simulink model "EV_dcm_sol"  (Simulink 7.1)
settings: Solver=ode4  StartTime=SIM.t_min  StopTime=SIM.t_simul  FixedStep=1e-3  RelTol=1e-3
undefined symbols (not defined in the file): BATp, CHAi, CHAp, CHp, EMi, EMp, MTp, RDp
libraries: simulink x1
settings Model: Creator=Tony  LastModifiedBy=Alain  ExtModeTrigMode=oneshot  ExtModeArmWhenConnect=off
settings DataIOCC: LimitDataPoints=off  SignalLoggingName=sigsOut
settings OptimizationCC: BooleanDataType=off  InitFltsAndDblsToZero=off
settings DebuggingCC: SaveWithParameterizedLinksMsg=none  SignalResolutionControl=TryResolveAllWithWarning  SolverPrmCheckMsg=none  MultiTaskDSMMsg=warning  MultiTaskCondExecSysMsg=none  StrictBusMsg=None
settings HardwareCC: TargetUnknown=on
settings RTWCC: IncludeERTFirstTime=on

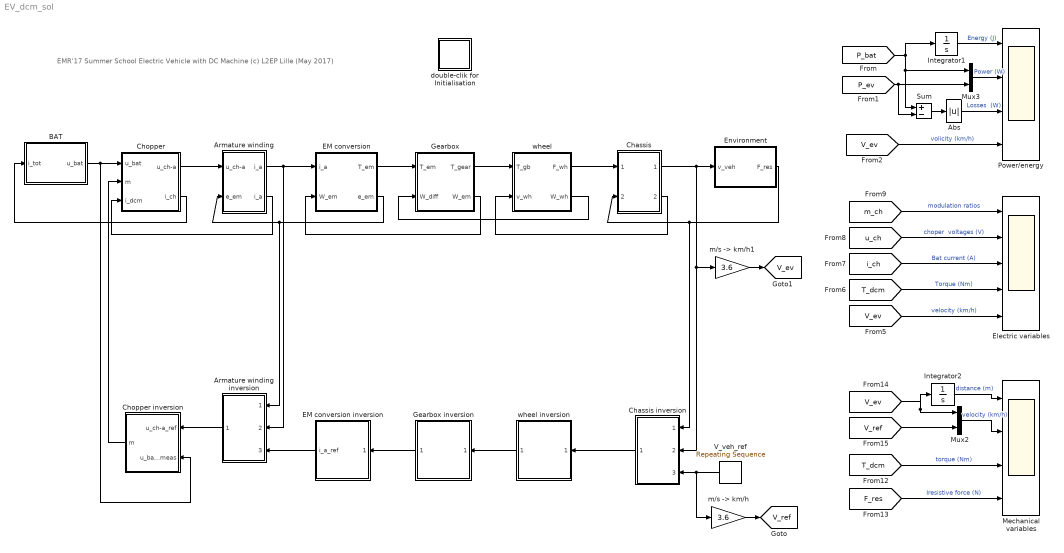
== system EV_dcm_sol ==
  note: EMR'17 Summer School
      | Electric Vehicle with DC Machine
      | (c) L2EP Lille (May 2017)
  Abs : Abs  OutDataType=sfix(16)  OutScaling=2^0
  Armature winding : Subsystem  AncestorBlock=simulink/REM/EA
      mask Type: CM
      mask Display: plot(0,0,100,100,[10,10,90,90,10],[90,10,10,90,90], [10,90],[10,90])
  Armature winding inversion : Subsystem  Orientation=left  AncestorBlock=simulink/SMC/Asservissement Correcteur IP
      mask Display: plot(0,0,100,100, [10,30,90,70,10,90],[90,10,10,90,90,10])
  BAT : Subsystem  AncestorBlock=simulink/REM/SE
      mask Display:
      | plot(0,0,100,100, 1.2*[50,57.68,60.77,63.08,64.97,66.58,68,69.26,70.4, 	71.42,72.36,78.28,80,78.28,72.36,71.42,70.4, 	69.26,68,66.58,64.97,63.08,60.77,57.68,50,42.32, 	39.23,36.92,35.03,33.42,32,30.74,29.6,28.58, 	27.64,21.72,20,21.72,27.64,28.58,29.6,30.74,32, 	33.42,35.03,36.92,39.23,42.32,50]-10, 1.2*[20,21,22,23,24,25,26,27,28,29,30,40,50,60,70,71,72, 	73,74,75,76,77,78,79,80,79,78,77,76,75,74,73,72, 	71,70,60,50,40,30,29,28,27,26,25,24,23,22,21,20]-10)
      | disp('BAT')
  Chassis : Subsystem  AncestorBlock=simulink/REM/EA
      mask Type: CM
      mask Display: plot(0,0,100,100,[10,10,90,90,10],[90,10,10,90,90], [10,90],[10,90])
  Chassis inversion : Subsystem  Orientation=left  AncestorBlock=simulink/SMC/Asservissement Correcteur IP
      mask Display: plot(0,0,100,100, [10,30,90,70,10,90],[90,10,10,90,90,10])
  Chopper : Subsystem  AncestorBlock=simulink/REM/EC Elec
      mask Type: Hacheur
      mask Display: plot(0,0,100,100,[10,10,90,90,10],[90,10,10,90,90])
  Chopper inversion : Subsystem  Orientation=left  AncestorBlock=simulink/SMC/Inversion EC avec mesure
      mask Display: plot(0,0,100,100,[10,30,90,70,10],[90,10,10,90,90])
  EM conversion : Subsystem  AncestorBlock=simulink/REM/EC EM
      mask Display: plot(0,0,100,100, 1.4*[50,57.68,60.77,63.08,64.97,66.58,68,69.26,70.4, 	71.42,72.36,78.28,80,78.28,72.36,71.42,70.4, 	69.26,68,66.58,64.97,63.08,60.77,57.68,50,42.32, 	39.23,36.92,35.03,33.42,32,30.74,29.6,28.58, 	27.64,21.72,20,21.72,27.64,28.58,29.6,30.74,32, 	33.42,35.03,36.92,39.23,42.32,50]-20, 1.4*[20,21,22,23,24,25,26,27,28,29,30,40,50,60,70,71,72, 	73,74,75,76,77,78,79,80,79,78,77,76,75,74,73,72, 	71,70,60,50,40,30,29,28,27,26,25,24,23,22,21,20]-20)
  EM conversion inversion : Subsystem  Orientation=left  AncestorBlock=simulink/SMC/Inversion EC avec mesure
      mask Display: plot(0,0,100,100,[10,30,90,70,10],[90,10,10,90,90])
  Electric variables : Scope  NumInputPorts=5
      settings: TimeRange=200  YMin=-0.5~-100~-20~-100~0  YMax=1~400~60~150~60  SaveName=ScopeData3  Decimation=10
  Environment : Subsystem  AncestorBlock=simulink/REM/SE
      mask Display:
      | plot(0,0,100,100, 1.2*[50,57.68,60.77,63.08,64.97,66.58,68,69.26,70.4, 	71.42,72.36,78.28,80,78.28,72.36,71.42,70.4, 	69.26,68,66.58,64.97,63.08,60.77,57.68,50,42.32, 	39.23,36.92,35.03,33.42,32,30.74,29.6,28.58, 	27.64,21.72,20,21.72,27.64,28.58,29.6,30.74,32, 	33.42,35.03,36.92,39.23,42.32,50]-10, 1.2*[20,21,22,23,24,25,26,27,28,29,30,40,50,60,70,71,72, 	73,74,75,76,77,78,79,80,79,78,77,76,75,74,73,72, 	71,70,60,50,40,30,29,28,27,26,25,24,23,22,21,20]-10)
      | disp('ROAD')
  Gearbox : Subsystem  AncestorBlock=simulink/REM/EC Elec
      mask Type: Hacheur
      mask Display: plot(0,0,100,100,[10,10,90,90,10],[90,10,10,90,90])
  Gearbox inversion : Subsystem  Orientation=left  AncestorBlock=simulink/SMC/Inversion EC avec mesure
      mask Display: plot(0,0,100,100,[10,30,90,70,10],[90,10,10,90,90])
  Integrator1 : Integrator
  Integrator2 : Integrator
  Mechanical variables : Scope  NumInputPorts=4
      settings: TimeRange=200  YMin=-1000~0~-100~0  YMax=4000~60~150~200  SaveName=ScopeData5  Decimation=10
  Mux2 : Mux  Inputs=2
  Mux3 : Mux  Inputs=2
  Power/energy : Scope  NumInputPorts=4
      settings: TimeRange=200  YMin=0~-10000~0~0  YMax=500000~20000~8000~60  Decimation=10
  Sum : Sum  Inputs=+-  OutDataType=sfix(16)  OutScaling=2^0  SaturateOnIntegerOverflow=on  InputSameDT=on  OutDataTypeStr=Inherit: Same as first input
  V_veh_ref : simulink/Sources/Repeating Sequence  Orientation=left  SystemSampleTime=-1  rep_seq_t=CYCL.time_ECE  rep_seq_y=CYCL.velocity_ECE
  double-clik for Initialisation : Subsystem
      settings: OpenFcn=init_EV_dcm_sol
      mask Type: Initialisation
      mask Display: disp('INIT')
  "m/s -> km/h" : Gain  Gain=3.6
  "m/s -> km/h1" : Gain  Gain=3.6
  wheel : Subsystem  AncestorBlock=simulink/REM/EC Elec
      mask Type: Hacheur
      mask Display: plot(0,0,100,100,[10,10,90,90,10],[90,10,10,90,90])
  wheel inversion : Subsystem  Orientation=left  AncestorBlock=simulink/SMC/Inversion EC avec mesure
      mask Display: plot(0,0,100,100,[10,30,90,70,10],[90,10,10,90,90])
  tag scope: V_ev=global, V_ref=global
  wires:
  BAT/1(u_bat) -> Chopper/1(u_bat), Chopper inversion/2(u_bat_meas)
  Chopper/2(i_ch) -> BAT/1(i_tot)
  Armature winding/2(i_a) -> Chopper/3(i_dcm)
  EM conversion/1(T_em) -> Gearbox/1(T_em)
  EM conversion/2(e_em) -> Armature winding/2(e_em), Armature winding inversion/1(e_em_meas)
  Gearbox/2(W_em) -> EM conversion/2(W_em)
  Chassis/1("v_veh ") -> Environment/1(v_veh), Chassis inversion/2(v_veh_meas), "m/s -> km/h1"/1
  V_veh_ref/1 -> Chassis inversion/3(v_veh_ref), "m/s -> km/h"/1
  Chassis inversion/1(F_veh_ref) -> wheel inversion/1(F_rwh_ref)
  wheel inversion/1(T_rdiff_ref) -> Gearbox inversion/1(T_gear_ref)
  Gearbox inversion/1(T_em_ref) -> EM conversion inversion/1(T_em_ref)
  Armature winding/1("i_a ") -> EM conversion/1(i_a), Armature winding inversion/2(i_a_meas)
  EM conversion inversion/1(i_a_ref) -> Armature winding inversion/3(i_a_ref)
  Chopper/1(u_ch-a) -> Armature winding/1(u_ch-a)
  Armature winding inversion/1(u_ch-a_ref) -> Chopper inversion/1(u_ch-a_ref)
  Chopper inversion/1(m) -> Chopper/2(m)
  [V_ev] -> Mux2/1, Integrator2/1
  [V_ref] -> Mux2/2
  Mux2/1 -> Mechanical variables/2  "velocity (km/h)"
  Integrator2/1 -> Mechanical variables/1  "distance (m)"
  [F_res] -> Mechanical variables/4  "Iresistive force (N)"
  [T_dcm] -> Mechanical variables/3  "torque (Nm)"
  "m/s -> km/h"/1 -> [V_ref]
  "m/s -> km/h1"/1 -> [V_ev]
  Sum/1 -> Abs/1
  [P_bat] -> Mux3/1, Sum/1, Integrator1/1
  [P_ev] -> Mux3/2, Sum/2
  [V_ev] -> Power/energy/4  "volicity (km/h)"
  Abs/1 -> Power/energy/3  "Losses  (W)"
  Mux3/1 -> Power/energy/2  "Power (W)"
  Integrator1/1 -> Power/energy/1  "Energy (J)"
  [V_ev] -> Electric variables/5  "velocity (km/h)"
  [T_dcm] -> Electric variables/4  "Torque (Nm)"
  [i_ch] -> Electric variables/3  "Bat current (A)"
  [u_ch] -> Electric variables/2  "choper  voltages (V)"
  [m_ch] -> Electric variables/1  "modulation ratios"
  Gearbox/1(T_gear) -> wheel/1(T_gb)
  wheel/1(F_wh) -> Chassis/1(F_wh)
  Chassis/2(v_veh) -> wheel/2(v_wh)
  wheel/2(W_wh) -> Gearbox/2(W_diff)
  Environment/1(F_res) -> Chassis/2(F_res), Chassis inversion/1(F_res_meas)

== system EV_dcm_sol/Armature winding ==
  u_ch-a : Inport
  e_em : Inport  Orientation=left  Port=2
  +/- : Sum  Inputs=+-  SaturateOnIntegerOverflow=on  InputSameDT=on  OutDataTypeStr=Inherit: Same as first input
  Transfer Fcn : TransferFcn  Numerator=[EMp.K_arm]  Denominator=[EMp.T_arm 1]
  "i_a " : Outport  InitialOutput=0
  i_a : Outport  Orientation=left  Port=2  InitialOutput=0
  wires:
  u_ch-a/1 -> +/-/1
  Transfer Fcn/1 -> i_a/1, "i_a "/1
  e_em/1 -> +/-/2
  +/-/1 -> Transfer Fcn/1

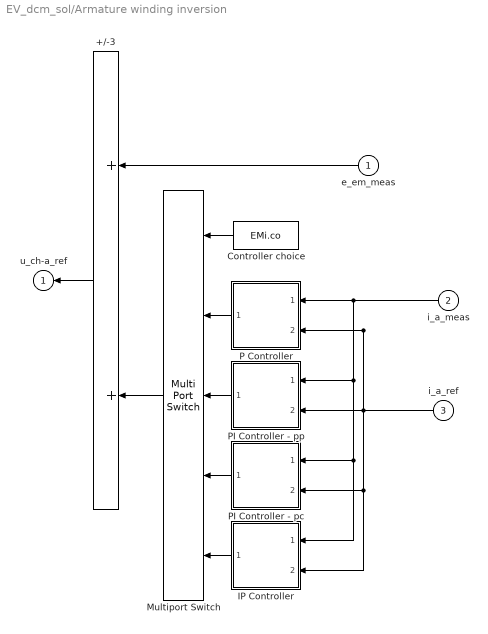
== system EV_dcm_sol/Armature winding inversion ==
  e_em_meas : Inport  Orientation=left
  i_a_meas : Inport  Orientation=left  Port=2
  i_a_ref : Inport  Orientation=left  Port=3
  +/-3 : Sum  Orientation=left  SaturateOnIntegerOverflow=on  InputSameDT=on  OutDataTypeStr=Inherit: Same as first input
  Controller choice : Constant  Orientation=left  Value=EMi.co
  IP Controller : Subsystem  Orientation=left
  Multiport Switch : MultiPortSwitch  Orientation=left  Inputs=4
  P Controller : Subsystem  Orientation=left
  PI Controller - pc : Subsystem  Orientation=left
  PI Controller - pp : Subsystem  Orientation=left
  u_ch-a_ref : Outport  Orientation=left  InitialOutput=0
  wires:
  Controller choice/1 -> Multiport Switch/1
  i_a_ref/1 -> PI Controller - pp/2(i_a_ref), PI Controller - pc/2(i_a_ref), IP Controller/2(i_a_ref), P Controller/2(i_a_ref)
  i_a_meas/1 -> PI Controller - pp/1(i_a_meas), PI Controller - pc/1(i_a_meas), IP Controller/1(i_a_meas), P Controller/1(i_a_meas)
  PI Controller - pc/1(u_ch-a_ref') -> Multiport Switch/4
  PI Controller - pp/1(u_ch-a_ref') -> Multiport Switch/3
  P Controller/1(u_ch-a_ref') -> Multiport Switch/2
  +/-3/1 -> u_ch-a_ref/1
  IP Controller/1(u_ch-a_ref') -> Multiport Switch/5
  Multiport Switch/1 -> +/-3/2
  e_em_meas/1 -> +/-3/1

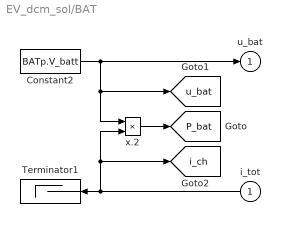
== system EV_dcm_sol/BAT ==
  i_tot : Inport  Orientation=left
  Constant2 : Constant  Value=BATp.V_batt
  Terminator1 : Terminator
  x.2 : Product  OutDataType=sfix(16)  OutScaling=2^0  SaturateOnIntegerOverflow=on  InputSameDT=on  OutDataTypeStr=Inherit: Same as first input
  u_bat : Outport  InitialOutput=0
  tag scope: P_bat=global, i_ch=global, u_bat=global
  wires:
  Constant2/1 -> u_bat/1, x.2/1, [u_bat]
  i_tot/1 -> Terminator1/1, x.2/2, [i_ch]
  x.2/1 -> [P_bat]

== system EV_dcm_sol/Chassis ==
  F_wh : Inport
  F_res : Inport  Orientation=left  Port=2
  +/- : Sum  Inputs=+-  SaturateOnIntegerOverflow=on  InputSameDT=on  OutDataTypeStr=Inherit: Same as first input
  Transfer Fcn : TransferFcn  Numerator=[CHAp.K_eq]  Denominator=[1 0]
  "v_veh " : Outport  InitialOutput=0
  v_veh : Outport  Orientation=left  Port=2  InitialOutput=0
  wires:
  +/-/1 -> Transfer Fcn/1
  F_res/1 -> +/-/2
  Transfer Fcn/1 -> "v_veh "/1, v_veh/1
  F_wh/1 -> +/-/1

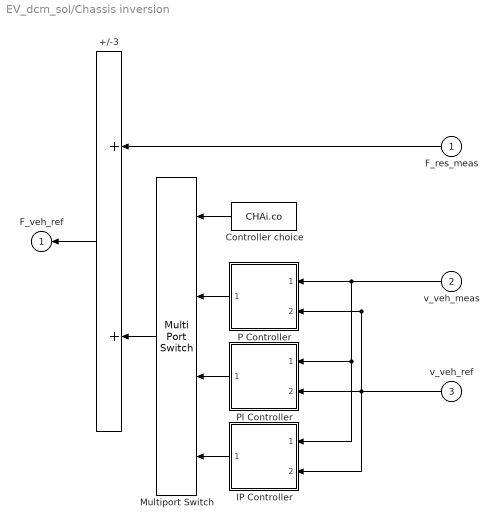
== system EV_dcm_sol/Chassis inversion ==
  F_res_meas : Inport  Orientation=left
  v_veh_meas : Inport  Orientation=left  Port=2
  v_veh_ref : Inport  Orientation=left  Port=3
  +/-3 : Sum  Orientation=left  SaturateOnIntegerOverflow=on  InputSameDT=on  OutDataTypeStr=Inherit: Same as first input
  Controller choice : Constant  Orientation=left  Value=CHAi.co
  IP Controller : Subsystem  Orientation=left
  Multiport Switch : MultiPortSwitch  Orientation=left
  P Controller : Subsystem  Orientation=left
  PI Controller : Subsystem  Orientation=left
  F_veh_ref : Outport  Orientation=left  InitialOutput=0
  wires:
  +/-3/1 -> F_veh_ref/1
  F_res_meas/1 -> +/-3/1
  Multiport Switch/1 -> +/-3/2
  P Controller/1(F_veh_ref') -> Multiport Switch/2
  PI Controller/1(F_veh_ref') -> Multiport Switch/3
  IP Controller/1(F_veh_ref') -> Multiport Switch/4
  v_veh_meas/1 -> P Controller/1(v_veh_meas), PI Controller/1(v_veh_meas), IP Controller/1(v_veh_meas)
  v_veh_ref/1 -> P Controller/2(v_veh_ref), PI Controller/2(v_veh_ref), IP Controller/2(v_veh_ref)
  Controller choice/1 -> Multiport Switch/1

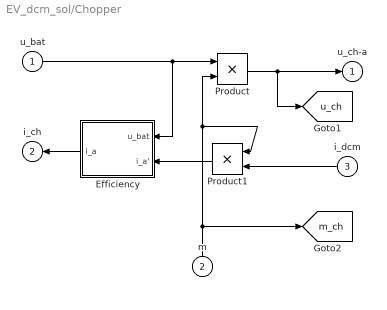
== system EV_dcm_sol/Chopper ==
  u_bat : Inport
  m : Inport  Orientation=up  Port=2
  i_dcm : Inport  Orientation=left  Port=3
  Efficiency : Subsystem  Orientation=left
  Product : Product  RndMeth=Zero
  Product1 : Product  Orientation=left  RndMeth=Zero
  u_ch-a : Outport  InitialOutput=0
  i_ch : Outport  Orientation=left  Port=2  InitialOutput=0
  tag scope: m_ch=global, u_ch=global
  wires:
  Product/1 -> u_ch-a/1, [u_ch]
  i_dcm/1 -> Product1/2
  m/1 -> Product1/1, Product/2, [m_ch]
  u_bat/1 -> Product/1, Efficiency/1(u_bat)
  Product1/1 -> Efficiency/2(i_a')
  Efficiency/1(i_a) -> i_ch/1

== system EV_dcm_sol/Chopper inversion ==
  u_ch-a_ref : Inport  Orientation=left
  u_bat_meas : Inport  Orientation=left  Port=2
  Divide : Product  Orientation=left  Inputs=*/
  Saturation : Saturate  Orientation=left  UpperLimit=1  LowerLimit=-1
  m : Outport  Orientation=left  InitialOutput=0
  wires:
  Divide/1 -> Saturation/1
  u_ch-a_ref/1 -> Divide/1
  u_bat_meas/1 -> Divide/2
  Saturation/1 -> m/1

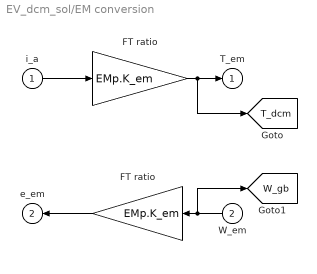
== system EV_dcm_sol/EM conversion ==
  i_a : Inport
  W_em : Inport  Orientation=left  Port=2
  FT ratio : Gain  Gain=EMp.K_em
  "FT ratio " : Gain  Orientation=left  Gain=EMp.K_em
  T_em : Outport  InitialOutput=0
  e_em : Outport  Orientation=left  Port=2  InitialOutput=0
  tag scope: T_dcm=global, W_gb=global
  wires:
  "FT ratio "/1 -> e_em/1
  i_a/1 -> FT ratio/1
  FT ratio/1 -> T_em/1, [T_dcm]
  W_em/1 -> "FT ratio "/1, [W_gb]

== system EV_dcm_sol/EM conversion inversion ==
  T_em_ref : Inport  Orientation=left
  "1/FT ratio " : Gain  Orientation=left  Gain=1/EMp.K_em
  i_a_ref : Outport  Orientation=left  InitialOutput=0
  wires:
  "1/FT ratio "/1 -> i_a_ref/1
  T_em_ref/1 -> "1/FT ratio "/1

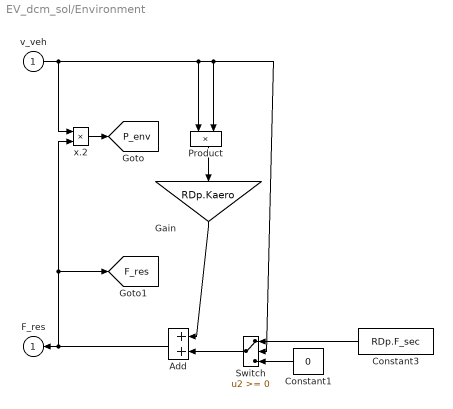
== system EV_dcm_sol/Environment ==
  v_veh : Inport
  Add : Sum  Orientation=left
  Constant1 : Constant  Orientation=left  Value=0
  Constant3 : Constant  Orientation=left  Value=RDp.F_sec
  Gain : Gain  Orientation=down  Gain=RDp.Kaero  SaturateOnIntegerOverflow=on  OutDataTypeStr=Inherit: Same as input  ParamDataTypeStr=Inherit: Same as input
  Product : Product  Orientation=down  SaturateOnIntegerOverflow=on  InputSameDT=on  OutDataTypeStr=Inherit: Same as first input
  Switch : Switch  Orientation=left
  x.2 : Product  OutDataType=sfix(16)  OutScaling=2^0  SaturateOnIntegerOverflow=on  InputSameDT=on  OutDataTypeStr=Inherit: Same as first input
  F_res : Outport  Orientation=left  InitialOutput=0
  tag scope: F_res=global, P_env=global
  wires:
  Product/1 -> Gain/1
  Gain/1 -> Add/1
  Add/1 -> F_res/1, x.2/2, [F_res]
  Constant1/1 -> Switch/3
  Constant3/1 -> Switch/1
  Switch/1 -> Add/2
  v_veh/1 -> Switch/2, Product/2, Product/1, x.2/1
  x.2/1 -> [P_env]

== system EV_dcm_sol/Gearbox ==
  T_em : Inport
  W_diff : Inport  Orientation=left  Port=2
  Efficiency : Subsystem
  FT ratio : Gain  Gain=MTp.K_gear
  "FT ratio " : Gain  Orientation=left  Gain=MTp.K_gear
  T_gear : Outport  InitialOutput=0
  W_em : Outport  Orientation=left  Port=2  InitialOutput=0
  wires:
  Efficiency/1(T_gear') -> FT ratio/1
  "FT ratio "/1 -> Efficiency/2(W_em), W_em/1
  T_em/1 -> Efficiency/1(T_em)
  FT ratio/1 -> T_gear/1
  W_diff/1 -> "FT ratio "/1

== system EV_dcm_sol/Gearbox inversion ==
  T_gear_ref : Inport  Orientation=left
  "1/FT ratio " : Gain  Orientation=left  Gain=1/MTp.K_gear
  T_em_ref : Outport  Orientation=left  InitialOutput=0
  wires:
  T_gear_ref/1 -> "1/FT ratio "/1
  "1/FT ratio "/1 -> T_em_ref/1

== system EV_dcm_sol/double-clik for Initialisation ==

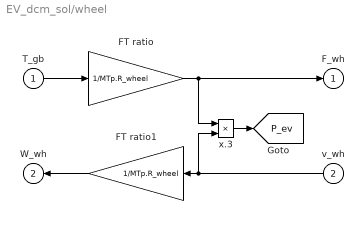
== system EV_dcm_sol/wheel ==
  T_gb : Inport
  v_wh : Inport  Orientation=left  Port=2
  FT ratio : Gain  Gain=1/MTp.R_wheel
  FT ratio1 : Gain  Orientation=left  Gain=1/MTp.R_wheel
  x.3 : Product  OutDataType=sfix(16)  OutScaling=2^0  SaturateOnIntegerOverflow=on  InputSameDT=on  OutDataTypeStr=Inherit: Same as first input
  F_wh : Outport  InitialOutput=0
  W_wh : Outport  Orientation=left  Port=2  InitialOutput=0
  tag scope: P_ev=global
  wires:
  v_wh/1 -> FT ratio1/1, x.3/2
  FT ratio/1 -> F_wh/1, x.3/1
  T_gb/1 -> FT ratio/1
  FT ratio1/1 -> W_wh/1
  x.3/1 -> [P_ev]

== system EV_dcm_sol/wheel inversion ==
  F_rwh_ref : Inport  Orientation=left
  "1/FT ratio " : Gain  Orientation=left  Gain=MTp.R_wheel
  T_rdiff_ref : Outport  Orientation=left  InitialOutput=0
  wires:
  "1/FT ratio "/1 -> T_rdiff_ref/1
  F_rwh_ref/1 -> "1/FT ratio "/1

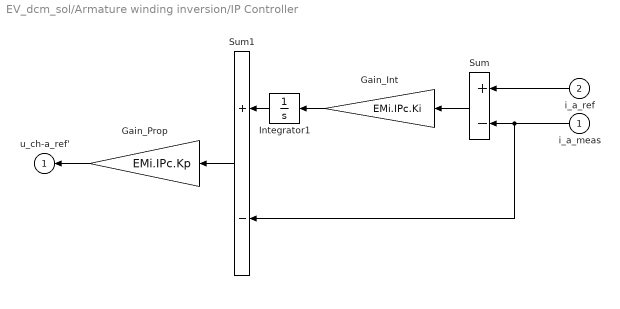
== system EV_dcm_sol/Armature winding inversion/IP Controller ==
  i_a_meas : Inport  Orientation=left
  i_a_ref : Inport  Orientation=left  Port=2
  Gain_Int : Gain  Orientation=left  Gain=EMi.IPc.Ki  SaturateOnIntegerOverflow=on  OutDataTypeStr=Inherit: Same as input  ParamDataTypeStr=Inherit: Same as input
  Gain_Prop : Gain  Orientation=left  Gain=EMi.IPc.Kp  SaturateOnIntegerOverflow=on  OutDataTypeStr=Inherit: Same as input  ParamDataTypeStr=Inherit: Same as input
  Integrator1 : Integrator  Orientation=left
  Sum : Sum  Orientation=left  Inputs=+-  SaturateOnIntegerOverflow=on  InputSameDT=on  OutDataTypeStr=Inherit: Same as first input
  Sum1 : Sum  Orientation=left  Inputs=+-  SaturateOnIntegerOverflow=on  InputSameDT=on  OutDataTypeStr=Inherit: Same as first input
  u_ch-a_ref' : Outport  Orientation=left  InitialOutput=0
  wires:
  i_a_ref/1 -> Sum/1
  i_a_meas/1 -> Sum1/2, Sum/2
  Gain_Int/1 -> Integrator1/1
  Sum/1 -> Gain_Int/1
  Sum1/1 -> Gain_Prop/1
  Integrator1/1 -> Sum1/1
  Gain_Prop/1 -> u_ch-a_ref'/1

== system EV_dcm_sol/Armature winding inversion/P Controller ==
  i_a_meas : Inport  Orientation=left
  i_a_ref : Inport  Orientation=left  Port=2
  Gain_Int : Gain  Orientation=left  Gain=EMi.Pc.Kp  SaturateOnIntegerOverflow=on  OutDataTypeStr=Inherit: Same as input  ParamDataTypeStr=Inherit: Same as input
  Sum : Sum  Orientation=left  Inputs=+-  SaturateOnIntegerOverflow=on  InputSameDT=on  OutDataTypeStr=Inherit: Same as first input
  u_ch-a_ref' : Outport  Orientation=left  InitialOutput=0
  wires:
  i_a_ref/1 -> Sum/1
  i_a_meas/1 -> Sum/2
  Gain_Int/1 -> u_ch-a_ref'/1
  Sum/1 -> Gain_Int/1

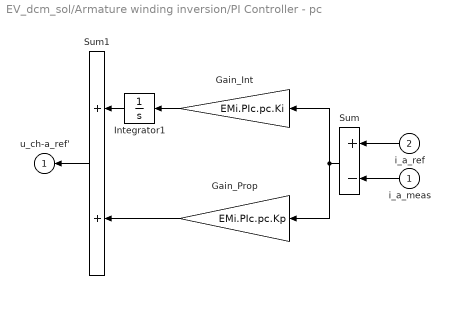
== system EV_dcm_sol/Armature winding inversion/PI Controller - pc ==
  i_a_meas : Inport  Orientation=left
  i_a_ref : Inport  Orientation=left  Port=2
  Gain_Int : Gain  Orientation=left  Gain=EMi.PIc.pc.Ki  SaturateOnIntegerOverflow=on  OutDataTypeStr=Inherit: Same as input  ParamDataTypeStr=Inherit: Same as input
  Gain_Prop : Gain  Orientation=left  Gain=EMi.PIc.pc.Kp  SaturateOnIntegerOverflow=on  OutDataTypeStr=Inherit: Same as input  ParamDataTypeStr=Inherit: Same as input
  Integrator1 : Integrator  Orientation=left
  Sum : Sum  Orientation=left  Inputs=+-  SaturateOnIntegerOverflow=on  InputSameDT=on  OutDataTypeStr=Inherit: Same as first input
  Sum1 : Sum  Orientation=left  SaturateOnIntegerOverflow=on  InputSameDT=on  OutDataTypeStr=Inherit: Same as first input
  u_ch-a_ref' : Outport  Orientation=left  InitialOutput=0
  wires:
  Integrator1/1 -> Sum1/1
  Sum1/1 -> u_ch-a_ref'/1
  Gain_Int/1 -> Integrator1/1
  i_a_meas/1 -> Sum/2
  i_a_ref/1 -> Sum/1
  Gain_Prop/1 -> Sum1/2
  Sum/1 -> Gain_Int/1, Gain_Prop/1

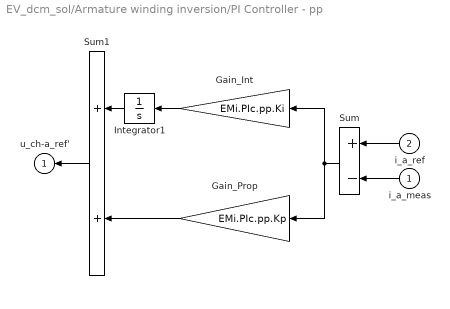
== system EV_dcm_sol/Armature winding inversion/PI Controller - pp ==
  i_a_meas : Inport  Orientation=left
  i_a_ref : Inport  Orientation=left  Port=2
  Gain_Int : Gain  Orientation=left  Gain=EMi.PIc.pp.Ki  SaturateOnIntegerOverflow=on  OutDataTypeStr=Inherit: Same as input  ParamDataTypeStr=Inherit: Same as input
  Gain_Prop : Gain  Orientation=left  Gain=EMi.PIc.pp.Kp  SaturateOnIntegerOverflow=on  OutDataTypeStr=Inherit: Same as input  ParamDataTypeStr=Inherit: Same as input
  Integrator1 : Integrator  Orientation=left
  Sum : Sum  Orientation=left  Inputs=+-  SaturateOnIntegerOverflow=on  InputSameDT=on  OutDataTypeStr=Inherit: Same as first input
  Sum1 : Sum  Orientation=left  SaturateOnIntegerOverflow=on  InputSameDT=on  OutDataTypeStr=Inherit: Same as first input
  u_ch-a_ref' : Outport  Orientation=left  InitialOutput=0
  wires:
  Sum/1 -> Gain_Prop/1, Gain_Int/1
  Gain_Prop/1 -> Sum1/2
  i_a_ref/1 -> Sum/1
  i_a_meas/1 -> Sum/2
  Gain_Int/1 -> Integrator1/1
  Sum1/1 -> u_ch-a_ref'/1
  Integrator1/1 -> Sum1/1

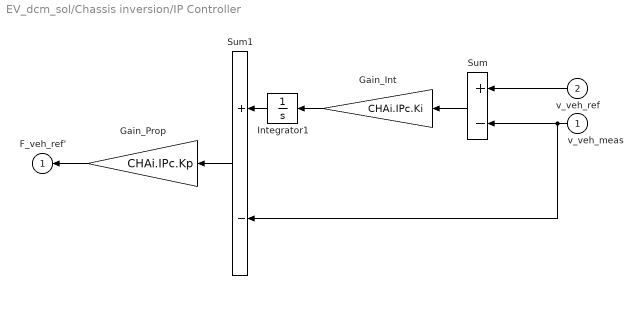
== system EV_dcm_sol/Chassis inversion/IP Controller ==
  v_veh_meas : Inport  Orientation=left
  v_veh_ref : Inport  Orientation=left  Port=2
  Gain_Int : Gain  Orientation=left  Gain=CHAi.IPc.Ki  SaturateOnIntegerOverflow=on  OutDataTypeStr=Inherit: Same as input  ParamDataTypeStr=Inherit: Same as input
  Gain_Prop : Gain  Orientation=left  Gain=CHAi.IPc.Kp  SaturateOnIntegerOverflow=on  OutDataTypeStr=Inherit: Same as input  ParamDataTypeStr=Inherit: Same as input
  Integrator1 : Integrator  Orientation=left
  Sum : Sum  Orientation=left  Inputs=+-  SaturateOnIntegerOverflow=on  InputSameDT=on  OutDataTypeStr=Inherit: Same as first input
  Sum1 : Sum  Orientation=left  Inputs=+-  SaturateOnIntegerOverflow=on  InputSameDT=on  OutDataTypeStr=Inherit: Same as first input
  F_veh_ref' : Outport  Orientation=left  InitialOutput=0
  wires:
  v_veh_ref/1 -> Sum/1
  v_veh_meas/1 -> Sum1/2, Sum/2
  Gain_Int/1 -> Integrator1/1
  Sum/1 -> Gain_Int/1
  Sum1/1 -> Gain_Prop/1
  Integrator1/1 -> Sum1/1
  Gain_Prop/1 -> F_veh_ref'/1

== system EV_dcm_sol/Chassis inversion/P Controller ==
  v_veh_meas : Inport  Orientation=left
  v_veh_ref : Inport  Orientation=left  Port=2
  Gain_Int : Gain  Orientation=left  Gain=CHAi.Pc.Kp  SaturateOnIntegerOverflow=on  OutDataTypeStr=Inherit: Same as input  ParamDataTypeStr=Inherit: Same as input
  Sum : Sum  Orientation=left  Inputs=+-  SaturateOnIntegerOverflow=on  InputSameDT=on  OutDataTypeStr=Inherit: Same as first input
  F_veh_ref' : Outport  Orientation=left  InitialOutput=0
  wires:
  Sum/1 -> Gain_Int/1
  Gain_Int/1 -> F_veh_ref'/1
  v_veh_meas/1 -> Sum/2
  v_veh_ref/1 -> Sum/1

== system EV_dcm_sol/Chassis inversion/PI Controller ==
  v_veh_meas : Inport  Orientation=left
  v_veh_ref : Inport  Orientation=left  Port=2
  Gain_Int : Gain  Orientation=left  Gain=CHAi.PIc.Ki  SaturateOnIntegerOverflow=on  OutDataTypeStr=Inherit: Same as input  ParamDataTypeStr=Inherit: Same as input
  Gain_Prop : Gain  Orientation=left  Gain=CHAi.PIc.Kp  SaturateOnIntegerOverflow=on  OutDataTypeStr=Inherit: Same as input  ParamDataTypeStr=Inherit: Same as input
  Integrator1 : Integrator  Orientation=left
  Sum : Sum  Orientation=left  Inputs=+-  SaturateOnIntegerOverflow=on  InputSameDT=on  OutDataTypeStr=Inherit: Same as first input
  Sum1 : Sum  Orientation=left  SaturateOnIntegerOverflow=on  InputSameDT=on  OutDataTypeStr=Inherit: Same as first input
  F_veh_ref' : Outport  Orientation=left  InitialOutput=0
  wires:
  Integrator1/1 -> Sum1/1
  Sum1/1 -> F_veh_ref'/1
  Gain_Int/1 -> Integrator1/1
  v_veh_meas/1 -> Sum/2
  v_veh_ref/1 -> Sum/1
  Gain_Prop/1 -> Sum1/2
  Sum/1 -> Gain_Int/1, Gain_Prop/1

== system EV_dcm_sol/Chopper/Efficiency ==
  u_bat : Inport  Orientation=left
  i_a' : Inport  Orientation=left  Port=2
  . : Product  Orientation=left  RndMeth=Zero
  Constant1 : Constant  Orientation=left  Value=CHp.eff
  Divide1 : Product  Orientation=left  Inputs=/*
  P_meca : Product  Orientation=left  RndMeth=Zero
  Switch : Switch  Orientation=left
  i_a : Outport  Orientation=left  InitialOutput=0
  wires:
  u_bat/1 -> P_meca/1
  i_a'/1 -> P_meca/2, Divide1/2, ./1
  Divide1/1 -> Switch/1
  ./1 -> Switch/3
  P_meca/1 -> Switch/2
  Switch/1 -> i_a/1
  Constant1/1 -> Divide1/1, ./2

== system EV_dcm_sol/Gearbox/Efficiency ==
  T_em : Inport
  W_em : Inport  Port=2
  " " : Product  RndMeth=Zero
  Constant1 : Constant  Value=MTp.Gear_eff
  Divide1 : Product  Inputs=*/
  P : Product  RndMeth=Zero
  Switch : Switch
  T_gear' : Outport  InitialOutput=0
  wires:
  Constant1/1 -> " "/1, Divide1/2
  P/1 -> Switch/2
  Switch/1 -> T_gear'/1
  Divide1/1 -> Switch/3
  " "/1 -> Switch/1
  W_em/1 -> P/2
  T_em/1 -> P/1, " "/2, Divide1/1
